simulink model "RCAM_MIMO_gain_testing"  (R2021b)
settings: Solver=VariableStepAuto  StartTime=0.0  StopTime=TF  FixedStep=0.0001  RelTol=1e-3
values from neighbouring files (symbols this model uses):
  A = rsys.A    [MIMO_synthesis.m]    (also in initializeConstantsMIMO.m = linear_sys.A; initializeConstantsMIMO_gain_testing.m = linear_sys.A)
  B = rsys.B    [MIMO_synthesis.m]    (also in initializeConstantsMIMO.m = linear_sys.B; initializeConstantsMIMO_gain_testing.m = linear_sys.B)
  C = rsys.C    [MIMO_synthesis.m]    (also in initializeConstantsMIMO.m = linear_sys.C; initializeConstantsMIMO_gain_testing.m = linear_sys.C)
  D = rsys.D    [MIMO_synthesis.m]    (also in initializeConstantsMIMO.m = linear_sys.D; initializeConstantsMIMO_gain_testing.m = linear_sys.D)
  k = k_gain.K    [initializeConstantsMIMO.m]    (also in initializeConstantsMIMO_gain_testing.m)
  x0 = [85 ... (first row only)    [initializeConstantsMIMO.m]    (also in initializeConstantsMIMO_gain_testing.m)
settings Model: Creator=khanh  LastModifiedBy=khanh

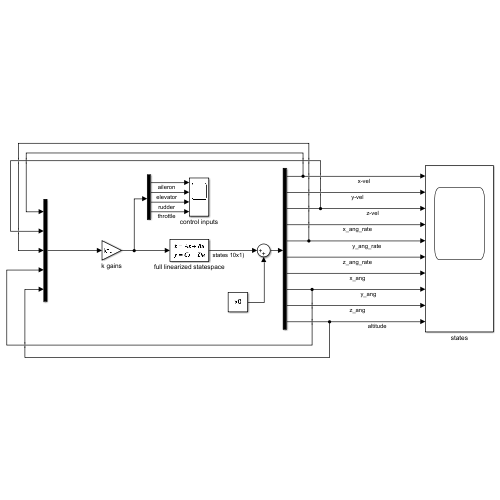
[thumbnail: Simulink's stored preview of the top-level diagram]
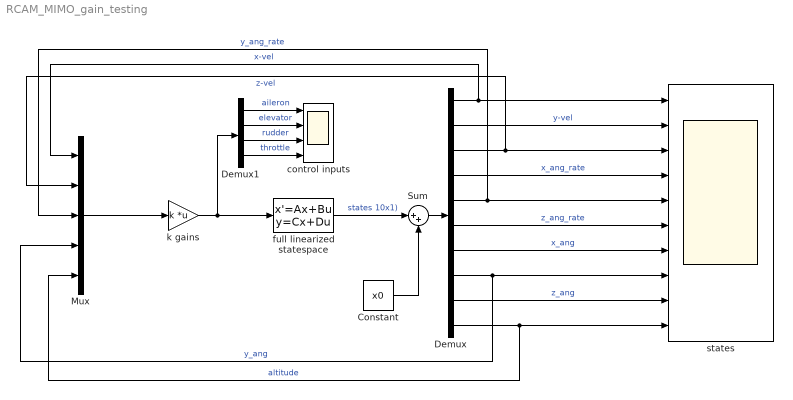
== system RCAM_MIMO_gain_testing ==
  Constant : Constant  Value=x0
  Demux : Demux  Outputs=10
  Demux1 : Demux
  Mux : Mux  Inputs=5
  Sum : Sum  Inputs=|++
  control inputs : Scope  NumInputPorts=4
  full linearized statespace : StateSpace  A=A  B=B  C=C  D=D  InitialCondition=0
  k gains : Gain  Gain=k  Multiplication=Matrix(K*u)
  states : Scope  NumInputPorts=10
  wires:
  k gains/1 -> Demux1/1, full linearized statespace/1
  full linearized statespace/1 -> Sum/1  "states 10x1)"
  Demux/1 -> Mux/1, states/1  "x-vel"
  Demux/2 -> states/2  "y-vel"
  Demux/3 -> Mux/2, states/3  "z-vel"
  Demux/4 -> states/4  "x_ang_rate"
  Demux/7 -> states/7  "x_ang"
  Demux/8 -> Mux/4, states/8  "y_ang"
  Demux/9 -> states/9  "z_ang"
  Demux/10 -> Mux/5, states/10  "altitude"
  Demux/5 -> Mux/3, states/5  "y_ang_rate"
  Demux/6 -> states/6  "z_ang_rate"
  Demux1/3 -> control inputs/3  "rudder"
  Demux1/1 -> control inputs/1  "aileron"
  Demux1/2 -> control inputs/2  "elevator"
  Demux1/4 -> control inputs/4  "throttle"
  Sum/1 -> Demux/1
  Constant/1 -> Sum/2
  Mux/1 -> k gains/1
